simulink model "PID_Real_Time_System"  (R2018b)
settings: Solver=FixedStepAuto  StartTime=0.0  StopTime=30  RelTol=1e-3  EnableMultiTasking=on
values from neighbouring files (symbols this model uses):
  h = 5e-3    (= 0.005)    [main.m]
  kd = 40    [main.m]
  ki = 180    [main.m]
  kp = 497    [main.m]
libraries: arduinolib x2
settings Model: ExtModeTrigDuration=2  Creator=fred  LastModifiedBy=root
settings OptimizationCC: EnhancedBackFolding=on  PassReuseOutputArgsAs=Individual arguments  MaxStackSize=64  OptimizeBlockOrder=speed  DifferentSizesBufferReuse=on  OptimizationCustomize=off
settings DebuggingCC: ParameterTunabilityLossMsg=error
settings HardwareCC: ProdBitPerInt=16  ProdBitPerPointer=16  ProdBitPerSizeT=16  ProdBitPerPtrDiffT=16  ProdLargestAtomicFloat=None  ProdWordSize=8  ProdHWDeviceType=Atmel->AVR  UseEmbeddedCoderFeatures=off
settings SFSimCC: MATLABDynamicMemAlloc=off
settings RTWCC: SystemTargetFile=ert.tlc  HardwareBoard=Arduino Mega 2560  TemplateMakefile=ert_default_tmf  GenerateReport=on  Toolchain=Arduino AVR  BuildConfiguration=Faster Runs  IncludeHyperlinkInReport=on  LaunchReport=on  GenerateTraceInfo=on  GenerateTraceReport=on  GenerateTraceReportSl=on  GenerateTraceReportSf=on  GenerateTraceReportEml=on
settings CodeAppCC: ForceParamTrailComments=on  IgnoreCustomStorageClasses=off  OperatorAnnotations=on  SimulinkDataObjDesc=on  SFDataObjDesc=on  InsertBlockDesc=on
settings ERTTargetCC: SupportContinuousTime=on  SupportNonInlinedSFcns=on  SupportVariableSizeSignals=on

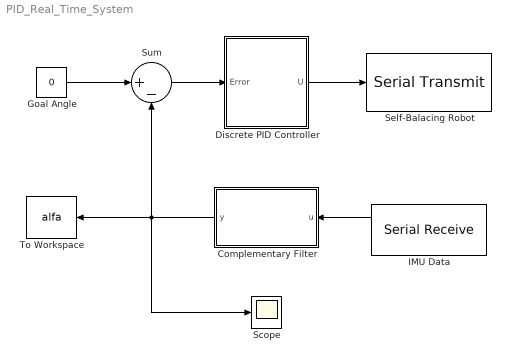
== system PID_Real_Time_System ==
  Complementary Filter : MATLAB Function  TreatAsAtomicUnit=on
  Discrete PID Controller : Subsystem
  Goal Angle : Constant  Value=0
  IMU Data : arduinolib/Serial Receive  isARMArch=off  portNumber=0  DataType=uint8  Datalength=1  SampleTime=h  showOutStatus=on  blockPlatform=arduino
      settings: SourceProductName=Simulink Support Package for Arduino Hardware  SourceProductBaseCode=ARDUINO
  Scope : Scope
  Self-Balacing Robot : arduinolib/Serial Transmit  portNumber=0  sendmode=write  sendformat=Decimal  floatprecision=2  blockPlatform=arduino
      settings: SourceProductName=Simulink Support Package for Arduino Hardware
  Sum : Sum  Inputs=|+-
  To Workspace : ToWorkspace  VariableName=alfa  SaveFormat=Timeseries  SampleTime=-1
      settings: Save2DSignal=2-D array (concatenate along first dimension)
  wires:
  Goal Angle/1 -> Sum/1
  Sum/1 -> Discrete PID Controller/1(Error)
  Discrete PID Controller/1(U) -> Self-Balacing Robot/1
  IMU Data/1 -> Complementary Filter/1(u)
  Complementary Filter/1(y) -> Scope/1, To Workspace/1, Sum/2

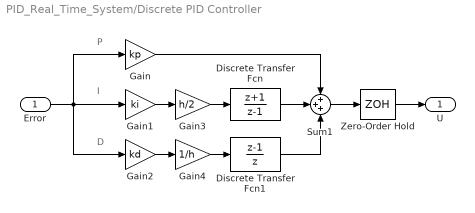
== system PID_Real_Time_System/Discrete PID Controller ==
  note: I
  note: D
  note: P
  Error : Inport
  Discrete Transfer Fcn : DiscreteTransferFcn  Numerator=[1 +1]  Denominator=[1 -1]  SampleTime=h
  Discrete Transfer Fcn1 : DiscreteTransferFcn  Numerator=[1 -1]  Denominator=[1 0]  SampleTime=h
  Gain : Gain  Gain=kp
  Gain1 : Gain  Gain=ki
  Gain2 : Gain  Gain=kd
  Gain3 : Gain  Gain=h/2
  Gain4 : Gain  Gain=1/h
  Sum1 : Sum  Inputs=+++
  Zero-Order Hold : ZeroOrderHold  SampleTime=h
  U : Outport
  wires:
  Gain1/1 -> Gain3/1
  Error/1 -> Gain1/1, Gain2/1, Gain/1
  Zero-Order Hold/1 -> U/1
  Sum1/1 -> Zero-Order Hold/1
  Gain2/1 -> Gain4/1
  Gain/1 -> Sum1/1
  Gain3/1 -> Discrete Transfer Fcn/1
  Discrete Transfer Fcn/1 -> Sum1/2
  Gain4/1 -> Discrete Transfer Fcn1/1
  Discrete Transfer Fcn1/1 -> Sum1/3

== matlab function PID_Real_Time_System/Complementary Filter ==
  data: u input; y output
function y = fcn(u)

y = u;
